simulink model "FM_Bistatic_Radar_Full"  (R2025a)
settings: Solver=VariableStepAuto  StartTime=0.0  StopTime=10.0  RelTol=1e-3
libraries: dspadpt3 x1, commanabbnd3 x1
(part 2 of 3)

== system FM_Bistatic_Radar_Full/Adaptive Filter/Gradiant Adaptive Lattice/50-Stage Lattice Predictor/Stage 41 ==
  note: K Update
  Forward Prediction Error : Inport
  Backward Prediction Error : Inport  Port=2
  K Input : Inport  Port=3
  Delay : Delay  DelayLength=1  InitialCondition=0
  K Update Equation : Subsystem
  Sum : Sum  Inputs=|++
  Sum1 : Sum  Inputs=|++
  Forward Prediction Error Output : Outport
  Backward Prediction Error Output : Outport  Port=2
  K : Outport  Port=3
  wires:
  Sum1/1 -> Backward Prediction Error Output/1
  Delay/1 -> Sum1/2, K Update Equation/2(B I/P)
  Sum/1 -> Forward Prediction Error Output/1
  K Update Equation/2(K) -> K/1, Sum1/1
  K Update Equation/1(*K (K conjugate)) -> Sum/2
  Backward Prediction Error/1 -> Delay/1
  Forward Prediction Error/1 -> Sum/1, K Update Equation/1(F I/P)
  K Input/1 -> K Update Equation/3(K I/P)

== system FM_Bistatic_Radar_Full/Adaptive Filter/Gradiant Adaptive Lattice/50-Stage Lattice Predictor/Stage 42 ==
  note: K Update
  Forward Prediction Error : Inport
  Backward Prediction Error : Inport  Port=2
  K Input : Inport  Port=3
  Delay : Delay  DelayLength=1  InitialCondition=0
  K Update Equation : Subsystem
  Sum : Sum  Inputs=|++
  Sum1 : Sum  Inputs=|++
  Forward Prediction Error Output : Outport
  Backward Prediction Error Output : Outport  Port=2
  K : Outport  Port=3
  wires:
  Sum1/1 -> Backward Prediction Error Output/1
  Delay/1 -> Sum1/2, K Update Equation/2(B I/P)
  Sum/1 -> Forward Prediction Error Output/1
  K Update Equation/2(K) -> K/1, Sum1/1
  K Update Equation/1(*K (K conjugate)) -> Sum/2
  Backward Prediction Error/1 -> Delay/1
  Forward Prediction Error/1 -> Sum/1, K Update Equation/1(F I/P)
  K Input/1 -> K Update Equation/3(K I/P)

== system FM_Bistatic_Radar_Full/Adaptive Filter/Gradiant Adaptive Lattice/50-Stage Lattice Predictor/Stage 43 ==
  note: K Update
  Forward Prediction Error : Inport
  Backward Prediction Error : Inport  Port=2
  K Input : Inport  Port=3
  Delay : Delay  DelayLength=1  InitialCondition=0
  K Update Equation : Subsystem
  Sum : Sum  Inputs=|++
  Sum1 : Sum  Inputs=|++
  Forward Prediction Error Output : Outport
  Backward Prediction Error Output : Outport  Port=2
  K : Outport  Port=3
  wires:
  Sum1/1 -> Backward Prediction Error Output/1
  Delay/1 -> Sum1/2, K Update Equation/2(B I/P)
  Sum/1 -> Forward Prediction Error Output/1
  K Update Equation/2(K) -> K/1, Sum1/1
  K Update Equation/1(*K (K conjugate)) -> Sum/2
  Backward Prediction Error/1 -> Delay/1
  Forward Prediction Error/1 -> Sum/1, K Update Equation/1(F I/P)
  K Input/1 -> K Update Equation/3(K I/P)

== system FM_Bistatic_Radar_Full/Adaptive Filter/Gradiant Adaptive Lattice/50-Stage Lattice Predictor/Stage 44 ==
  note: K Update
  Forward Prediction Error : Inport
  Backward Prediction Error : Inport  Port=2
  K Input : Inport  Port=3
  Delay : Delay  DelayLength=1  InitialCondition=0
  K Update Equation : Subsystem
  Sum : Sum  Inputs=|++
  Sum1 : Sum  Inputs=|++
  Forward Prediction Error Output : Outport
  Backward Prediction Error Output : Outport  Port=2
  K : Outport  Port=3
  wires:
  Sum1/1 -> Backward Prediction Error Output/1
  Delay/1 -> Sum1/2, K Update Equation/2(B I/P)
  Sum/1 -> Forward Prediction Error Output/1
  K Update Equation/2(K) -> K/1, Sum1/1
  K Update Equation/1(*K (K conjugate)) -> Sum/2
  Backward Prediction Error/1 -> Delay/1
  Forward Prediction Error/1 -> Sum/1, K Update Equation/1(F I/P)
  K Input/1 -> K Update Equation/3(K I/P)

== system FM_Bistatic_Radar_Full/Adaptive Filter/Gradiant Adaptive Lattice/50-Stage Lattice Predictor/Stage 45 ==
  note: K Update
  Forward Prediction Error : Inport
  Backward Prediction Error : Inport  Port=2
  K Input : Inport  Port=3
  Delay : Delay  DelayLength=1  InitialCondition=0
  K Update Equation : Subsystem
  Sum : Sum  Inputs=|++
  Sum1 : Sum  Inputs=|++
  Forward Prediction Error Output : Outport
  Backward Prediction Error Output : Outport  Port=2
  K : Outport  Port=3
  wires:
  Sum1/1 -> Backward Prediction Error Output/1
  Delay/1 -> Sum1/2, K Update Equation/2(B I/P)
  Sum/1 -> Forward Prediction Error Output/1
  K Update Equation/2(K) -> K/1, Sum1/1
  K Update Equation/1(*K (K conjugate)) -> Sum/2
  Backward Prediction Error/1 -> Delay/1
  Forward Prediction Error/1 -> Sum/1, K Update Equation/1(F I/P)
  K Input/1 -> K Update Equation/3(K I/P)

== system FM_Bistatic_Radar_Full/Adaptive Filter/Gradiant Adaptive Lattice/50-Stage Lattice Predictor/Stage 46 ==
  note: K Update
  Forward Prediction Error : Inport
  Backward Prediction Error : Inport  Port=2
  K Input : Inport  Port=3
  Delay : Delay  DelayLength=1  InitialCondition=0
  K Update Equation : Subsystem
  Sum : Sum  Inputs=|++
  Sum1 : Sum  Inputs=|++
  Forward Prediction Error Output : Outport
  Backward Prediction Error Output : Outport  Port=2
  K : Outport  Port=3
  wires:
  Sum1/1 -> Backward Prediction Error Output/1
  Delay/1 -> Sum1/2, K Update Equation/2(B I/P)
  Sum/1 -> Forward Prediction Error Output/1
  K Update Equation/2(K) -> K/1, Sum1/1
  K Update Equation/1(*K (K conjugate)) -> Sum/2
  Backward Prediction Error/1 -> Delay/1
  Forward Prediction Error/1 -> Sum/1, K Update Equation/1(F I/P)
  K Input/1 -> K Update Equation/3(K I/P)

== system FM_Bistatic_Radar_Full/Adaptive Filter/Gradiant Adaptive Lattice/50-Stage Lattice Predictor/Stage 47 ==
  note: K Update
  Forward Prediction Error : Inport
  Backward Prediction Error : Inport  Port=2
  K Input : Inport  Port=3
  Delay : Delay  DelayLength=1  InitialCondition=0
  K Update Equation : Subsystem
  Sum : Sum  Inputs=|++
  Sum1 : Sum  Inputs=|++
  Forward Prediction Error Output : Outport
  Backward Prediction Error Output : Outport  Port=2
  K : Outport  Port=3
  wires:
  Sum1/1 -> Backward Prediction Error Output/1
  Delay/1 -> Sum1/2, K Update Equation/2(B I/P)
  Sum/1 -> Forward Prediction Error Output/1
  K Update Equation/2(K) -> K/1, Sum1/1
  K Update Equation/1(*K (K conjugate)) -> Sum/2
  Backward Prediction Error/1 -> Delay/1
  Forward Prediction Error/1 -> Sum/1, K Update Equation/1(F I/P)
  K Input/1 -> K Update Equation/3(K I/P)

== system FM_Bistatic_Radar_Full/Adaptive Filter/Gradiant Adaptive Lattice/50-Stage Lattice Predictor/Stage 48 ==
  note: K Update
  Forward Prediction Error : Inport
  Backward Prediction Error : Inport  Port=2
  K Input : Inport  Port=3
  Delay : Delay  DelayLength=1  InitialCondition=0
  K Update Equation : Subsystem
  Sum : Sum  Inputs=|++
  Sum1 : Sum  Inputs=|++
  Forward Prediction Error Output : Outport
  Backward Prediction Error Output : Outport  Port=2
  K : Outport  Port=3
  wires:
  Sum1/1 -> Backward Prediction Error Output/1
  Delay/1 -> Sum1/2, K Update Equation/2(B I/P)
  Sum/1 -> Forward Prediction Error Output/1
  K Update Equation/2(K) -> K/1, Sum1/1
  K Update Equation/1(*K (K conjugate)) -> Sum/2
  Backward Prediction Error/1 -> Delay/1
  Forward Prediction Error/1 -> Sum/1, K Update Equation/1(F I/P)
  K Input/1 -> K Update Equation/3(K I/P)

== system FM_Bistatic_Radar_Full/Adaptive Filter/Gradiant Adaptive Lattice/50-Stage Lattice Predictor/Stage 49 ==
  note: K Update
  Forward Prediction Error : Inport
  Backward Prediction Error : Inport  Port=2
  K Input : Inport  Port=3
  Delay : Delay  DelayLength=1  InitialCondition=0
  K Update Equation : Subsystem
  Sum : Sum  Inputs=|++
  Sum1 : Sum  Inputs=|++
  Forward Prediction Error Output : Outport
  Backward Prediction Error Output : Outport  Port=2
  K : Outport  Port=3
  wires:
  Sum1/1 -> Backward Prediction Error Output/1
  Delay/1 -> Sum1/2, K Update Equation/2(B I/P)
  Sum/1 -> Forward Prediction Error Output/1
  K Update Equation/2(K) -> K/1, Sum1/1
  K Update Equation/1(*K (K conjugate)) -> Sum/2
  Backward Prediction Error/1 -> Delay/1
  Forward Prediction Error/1 -> Sum/1, K Update Equation/1(F I/P)
  K Input/1 -> K Update Equation/3(K I/P)

== system FM_Bistatic_Radar_Full/Adaptive Filter/Gradiant Adaptive Lattice/50-Stage Lattice Predictor/Stage 5 ==
  note: K Update
  Forward Prediction Error : Inport
  Backward Prediction Error : Inport  Port=2
  K Input : Inport  Port=3
  Delay : Delay  DelayLength=1  InitialCondition=0
  K Update Equation : Subsystem
  Sum : Sum  Inputs=|++
  Sum1 : Sum  Inputs=|++
  Forward Prediction Error Output : Outport
  Backward Prediction Error Output : Outport  Port=2
  K : Outport  Port=3
  wires:
  Sum1/1 -> Backward Prediction Error Output/1
  Delay/1 -> Sum1/2, K Update Equation/2(B I/P)
  Sum/1 -> Forward Prediction Error Output/1
  K Update Equation/2(K) -> K/1, Sum1/1
  K Update Equation/1(*K (K conjugate)) -> Sum/2
  Backward Prediction Error/1 -> Delay/1
  Forward Prediction Error/1 -> Sum/1, K Update Equation/1(F I/P)
  K Input/1 -> K Update Equation/3(K I/P)

== system FM_Bistatic_Radar_Full/Adaptive Filter/Gradiant Adaptive Lattice/50-Stage Lattice Predictor/Stage 50 ==
  note: K Update
  Forward Prediction Error : Inport
  Backward Prediction Error : Inport  Port=2
  K Input : Inport  Port=3
  Delay : Delay  DelayLength=1  InitialCondition=0
  K Update Equation : Subsystem
  Sum : Sum  Inputs=|++
  Sum1 : Sum  Inputs=|++
  Forward Prediction Error Output : Outport
  Backward Prediction Error Output : Outport  Port=2
  K : Outport  Port=3
  wires:
  Sum1/1 -> Backward Prediction Error Output/1
  Delay/1 -> Sum1/2, K Update Equation/2(B I/P)
  Sum/1 -> Forward Prediction Error Output/1
  K Update Equation/2(K) -> K/1, Sum1/1
  K Update Equation/1(*K (K conjugate)) -> Sum/2
  Backward Prediction Error/1 -> Delay/1
  Forward Prediction Error/1 -> Sum/1, K Update Equation/1(F I/P)
  K Input/1 -> K Update Equation/3(K I/P)

== system FM_Bistatic_Radar_Full/Adaptive Filter/Gradiant Adaptive Lattice/50-Stage Lattice Predictor/Stage 51 ==
  note: K Update
  Forward Prediction Error : Inport
  Backward Prediction Error : Inport  Port=2
  K Input : Inport  Port=3
  Delay : Delay  DelayLength=1  InitialCondition=0
  K Update Equation : Subsystem
  Sum : Sum  Inputs=|++
  Sum1 : Sum  Inputs=|++
  Forward Prediction Error Output : Outport
  Backward Prediction Error Output : Outport  Port=2
  K : Outport  Port=3
  wires:
  Sum1/1 -> Backward Prediction Error Output/1
  Delay/1 -> Sum1/2, K Update Equation/2(B I/P)
  Sum/1 -> Forward Prediction Error Output/1
  K Update Equation/2(K) -> K/1, Sum1/1
  K Update Equation/1(*K (K conjugate)) -> Sum/2
  Backward Prediction Error/1 -> Delay/1
  Forward Prediction Error/1 -> Sum/1, K Update Equation/1(F I/P)
  K Input/1 -> K Update Equation/3(K I/P)

== system FM_Bistatic_Radar_Full/Adaptive Filter/Gradiant Adaptive Lattice/50-Stage Lattice Predictor/Stage 6 ==
  note: K Update
  Forward Prediction Error : Inport
  Backward Prediction Error : Inport  Port=2
  K Input : Inport  Port=3
  Delay : Delay  DelayLength=1  InitialCondition=0
  K Update Equation : Subsystem
  Sum : Sum  Inputs=|++
  Sum1 : Sum  Inputs=|++
  Forward Prediction Error Output : Outport
  Backward Prediction Error Output : Outport  Port=2
  K : Outport  Port=3
  wires:
  Sum1/1 -> Backward Prediction Error Output/1
  Delay/1 -> Sum1/2, K Update Equation/2(B I/P)
  Sum/1 -> Forward Prediction Error Output/1
  K Update Equation/2(K) -> K/1, Sum1/1
  K Update Equation/1(*K (K conjugate)) -> Sum/2
  Backward Prediction Error/1 -> Delay/1
  Forward Prediction Error/1 -> Sum/1, K Update Equation/1(F I/P)
  K Input/1 -> K Update Equation/3(K I/P)

== system FM_Bistatic_Radar_Full/Adaptive Filter/Gradiant Adaptive Lattice/50-Stage Lattice Predictor/Stage 7 ==
  note: K Update
  Forward Prediction Error : Inport
  Backward Prediction Error : Inport  Port=2
  K Input : Inport  Port=3
  Delay : Delay  DelayLength=1  InitialCondition=0
  K Update Equation : Subsystem
  Sum : Sum  Inputs=|++
  Sum1 : Sum  Inputs=|++
  Forward Prediction Error Output : Outport
  Backward Prediction Error Output : Outport  Port=2
  K : Outport  Port=3
  wires:
  Sum1/1 -> Backward Prediction Error Output/1
  Delay/1 -> Sum1/2, K Update Equation/2(B I/P)
  Sum/1 -> Forward Prediction Error Output/1
  K Update Equation/2(K) -> K/1, Sum1/1
  K Update Equation/1(*K (K conjugate)) -> Sum/2
  Backward Prediction Error/1 -> Delay/1
  Forward Prediction Error/1 -> Sum/1, K Update Equation/1(F I/P)
  K Input/1 -> K Update Equation/3(K I/P)

== system FM_Bistatic_Radar_Full/Adaptive Filter/Gradiant Adaptive Lattice/50-Stage Lattice Predictor/Stage 8 ==
  note: K Update
  Forward Prediction Error : Inport
  Backward Prediction Error : Inport  Port=2
  K Input : Inport  Port=3
  Delay : Delay  DelayLength=1  InitialCondition=0
  K Update Equation : Subsystem
  Sum : Sum  Inputs=|++
  Sum1 : Sum  Inputs=|++
  Forward Prediction Error Output : Outport
  Backward Prediction Error Output : Outport  Port=2
  K : Outport  Port=3
  wires:
  Sum1/1 -> Backward Prediction Error Output/1
  Delay/1 -> Sum1/2, K Update Equation/2(B I/P)
  Sum/1 -> Forward Prediction Error Output/1
  K Update Equation/2(K) -> K/1, Sum1/1
  K Update Equation/1(*K (K conjugate)) -> Sum/2
  Backward Prediction Error/1 -> Delay/1
  Forward Prediction Error/1 -> Sum/1, K Update Equation/1(F I/P)
  K Input/1 -> K Update Equation/3(K I/P)

== system FM_Bistatic_Radar_Full/Adaptive Filter/Gradiant Adaptive Lattice/50-Stage Lattice Predictor/Stage 9 ==
  note: K Update
  Forward Prediction Error : Inport
  Backward Prediction Error : Inport  Port=2
  K Input : Inport  Port=3
  Delay : Delay  DelayLength=1  InitialCondition=0
  K Update Equation : Subsystem
  Sum : Sum  Inputs=|++
  Sum1 : Sum  Inputs=|++
  Forward Prediction Error Output : Outport
  Backward Prediction Error Output : Outport  Port=2
  K : Outport  Port=3
  wires:
  Sum1/1 -> Backward Prediction Error Output/1
  Delay/1 -> Sum1/2, K Update Equation/2(B I/P)
  Sum/1 -> Forward Prediction Error Output/1
  K Update Equation/2(K) -> K/1, Sum1/1
  K Update Equation/1(*K (K conjugate)) -> Sum/2
  Backward Prediction Error/1 -> Delay/1
  Forward Prediction Error/1 -> Sum/1, K Update Equation/1(F I/P)
  K Input/1 -> K Update Equation/3(K I/P)

== system FM_Bistatic_Radar_Full/Adaptive Filter/Gradiant Adaptive Lattice/50-Stage Lattice Predictor/Stage 1/K Update Equation ==
  F I/P : Inport
  B I/P : Inport  Port=2
  Conjugate : Math  Operator=conj  SignedPower=on  RndMeth=Zero
  Conjugate1 : Math  Operator=conj  SignedPower=on  RndMeth=Zero
  Constant : Constant  Value=0.01
  Dot Product : DotProduct  OutDataTypeStr=Inherit: Inherit via internal rule
  Dot Product1 : DotProduct  OutDataTypeStr=Inherit: Inherit via internal rule
  Subtract : Sum  Inputs=+-
  *K (K conjugate) : Outport
  K : Outport  Port=2
  wires:
  F I/P/1 -> Subtract/1, Dot Product/1
  B I/P/1 -> Conjugate/1
  Conjugate/1 -> Dot Product/2
  Constant/1 -> Dot Product1/2
  Dot Product/1 -> Dot Product1/1
  Conjugate1/1 -> *K (K conjugate)/1
  Dot Product1/1 -> Subtract/2
  Subtract/1 -> K/1, Conjugate1/1

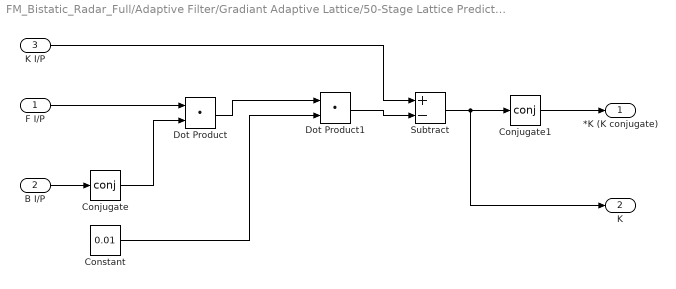
== system FM_Bistatic_Radar_Full/Adaptive Filter/Gradiant Adaptive Lattice/50-Stage Lattice Predictor/Stage 10/K Update Equation ==
  F I/P : Inport
  B I/P : Inport  Port=2
  K I/P : Inport  Port=3
  Conjugate : Math  Operator=conj  SignedPower=on  RndMeth=Zero
  Conjugate1 : Math  Operator=conj  SignedPower=on  RndMeth=Zero
  Constant : Constant  Value=0.01
  Dot Product : DotProduct  OutDataTypeStr=Inherit: Inherit via internal rule
  Dot Product1 : DotProduct  OutDataTypeStr=Inherit: Inherit via internal rule
  Subtract : Sum  Inputs=+-
  *K (K conjugate) : Outport
  K : Outport  Port=2
  wires:
  F I/P/1 -> Dot Product/1
  B I/P/1 -> Conjugate/1
  Conjugate/1 -> Dot Product/2
  Constant/1 -> Dot Product1/2
  Dot Product/1 -> Dot Product1/1
  Conjugate1/1 -> *K (K conjugate)/1
  Dot Product1/1 -> Subtract/2
  Subtract/1 -> K/1, Conjugate1/1
  K I/P/1 -> Subtract/1

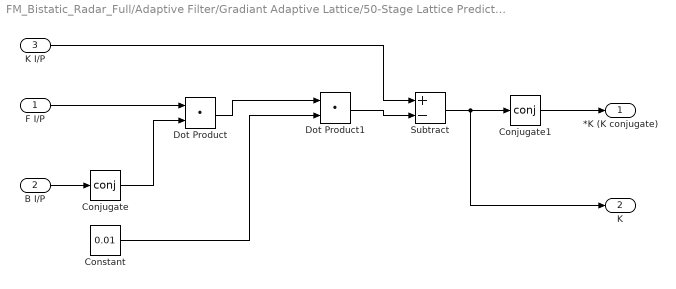
== system FM_Bistatic_Radar_Full/Adaptive Filter/Gradiant Adaptive Lattice/50-Stage Lattice Predictor/Stage 11/K Update Equation ==
  F I/P : Inport
  B I/P : Inport  Port=2
  K I/P : Inport  Port=3
  Conjugate : Math  Operator=conj  SignedPower=on  RndMeth=Zero
  Conjugate1 : Math  Operator=conj  SignedPower=on  RndMeth=Zero
  Constant : Constant  Value=0.01
  Dot Product : DotProduct  OutDataTypeStr=Inherit: Inherit via internal rule
  Dot Product1 : DotProduct  OutDataTypeStr=Inherit: Inherit via internal rule
  Subtract : Sum  Inputs=+-
  *K (K conjugate) : Outport
  K : Outport  Port=2
  wires:
  F I/P/1 -> Dot Product/1
  B I/P/1 -> Conjugate/1
  Conjugate/1 -> Dot Product/2
  Constant/1 -> Dot Product1/2
  Dot Product/1 -> Dot Product1/1
  Conjugate1/1 -> *K (K conjugate)/1
  Dot Product1/1 -> Subtract/2
  Subtract/1 -> K/1, Conjugate1/1
  K I/P/1 -> Subtract/1

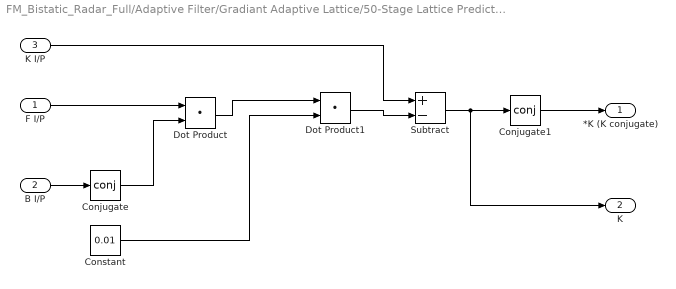
== system FM_Bistatic_Radar_Full/Adaptive Filter/Gradiant Adaptive Lattice/50-Stage Lattice Predictor/Stage 12/K Update Equation ==
  F I/P : Inport
  B I/P : Inport  Port=2
  K I/P : Inport  Port=3
  Conjugate : Math  Operator=conj  SignedPower=on  RndMeth=Zero
  Conjugate1 : Math  Operator=conj  SignedPower=on  RndMeth=Zero
  Constant : Constant  Value=0.01
  Dot Product : DotProduct  OutDataTypeStr=Inherit: Inherit via internal rule
  Dot Product1 : DotProduct  OutDataTypeStr=Inherit: Inherit via internal rule
  Subtract : Sum  Inputs=+-
  *K (K conjugate) : Outport
  K : Outport  Port=2
  wires:
  F I/P/1 -> Dot Product/1
  B I/P/1 -> Conjugate/1
  Conjugate/1 -> Dot Product/2
  Constant/1 -> Dot Product1/2
  Dot Product/1 -> Dot Product1/1
  Conjugate1/1 -> *K (K conjugate)/1
  Dot Product1/1 -> Subtract/2
  Subtract/1 -> K/1, Conjugate1/1
  K I/P/1 -> Subtract/1

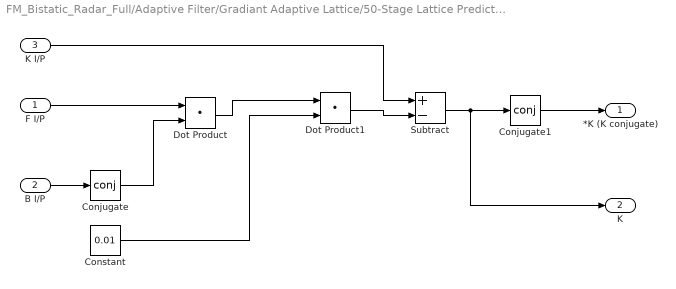
== system FM_Bistatic_Radar_Full/Adaptive Filter/Gradiant Adaptive Lattice/50-Stage Lattice Predictor/Stage 13/K Update Equation ==
  F I/P : Inport
  B I/P : Inport  Port=2
  K I/P : Inport  Port=3
  Conjugate : Math  Operator=conj  SignedPower=on  RndMeth=Zero
  Conjugate1 : Math  Operator=conj  SignedPower=on  RndMeth=Zero
  Constant : Constant  Value=0.01
  Dot Product : DotProduct  OutDataTypeStr=Inherit: Inherit via internal rule
  Dot Product1 : DotProduct  OutDataTypeStr=Inherit: Inherit via internal rule
  Subtract : Sum  Inputs=+-
  *K (K conjugate) : Outport
  K : Outport  Port=2
  wires:
  F I/P/1 -> Dot Product/1
  B I/P/1 -> Conjugate/1
  Conjugate/1 -> Dot Product/2
  Constant/1 -> Dot Product1/2
  Dot Product/1 -> Dot Product1/1
  Conjugate1/1 -> *K (K conjugate)/1
  Dot Product1/1 -> Subtract/2
  Subtract/1 -> K/1, Conjugate1/1
  K I/P/1 -> Subtract/1

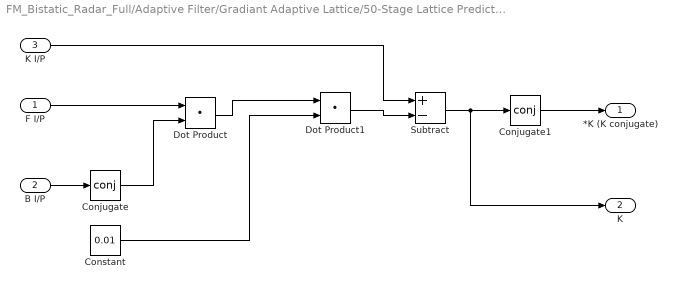
== system FM_Bistatic_Radar_Full/Adaptive Filter/Gradiant Adaptive Lattice/50-Stage Lattice Predictor/Stage 14/K Update Equation ==
  F I/P : Inport
  B I/P : Inport  Port=2
  K I/P : Inport  Port=3
  Conjugate : Math  Operator=conj  SignedPower=on  RndMeth=Zero
  Conjugate1 : Math  Operator=conj  SignedPower=on  RndMeth=Zero
  Constant : Constant  Value=0.01
  Dot Product : DotProduct  OutDataTypeStr=Inherit: Inherit via internal rule
  Dot Product1 : DotProduct  OutDataTypeStr=Inherit: Inherit via internal rule
  Subtract : Sum  Inputs=+-
  *K (K conjugate) : Outport
  K : Outport  Port=2
  wires:
  F I/P/1 -> Dot Product/1
  B I/P/1 -> Conjugate/1
  Conjugate/1 -> Dot Product/2
  Constant/1 -> Dot Product1/2
  Dot Product/1 -> Dot Product1/1
  Conjugate1/1 -> *K (K conjugate)/1
  Dot Product1/1 -> Subtract/2
  Subtract/1 -> K/1, Conjugate1/1
  K I/P/1 -> Subtract/1

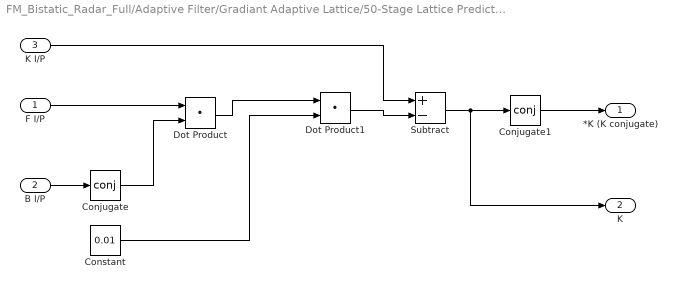
== system FM_Bistatic_Radar_Full/Adaptive Filter/Gradiant Adaptive Lattice/50-Stage Lattice Predictor/Stage 15/K Update Equation ==
  F I/P : Inport
  B I/P : Inport  Port=2
  K I/P : Inport  Port=3
  Conjugate : Math  Operator=conj  SignedPower=on  RndMeth=Zero
  Conjugate1 : Math  Operator=conj  SignedPower=on  RndMeth=Zero
  Constant : Constant  Value=0.01
  Dot Product : DotProduct  OutDataTypeStr=Inherit: Inherit via internal rule
  Dot Product1 : DotProduct  OutDataTypeStr=Inherit: Inherit via internal rule
  Subtract : Sum  Inputs=+-
  *K (K conjugate) : Outport
  K : Outport  Port=2
  wires:
  F I/P/1 -> Dot Product/1
  B I/P/1 -> Conjugate/1
  Conjugate/1 -> Dot Product/2
  Constant/1 -> Dot Product1/2
  Dot Product/1 -> Dot Product1/1
  Conjugate1/1 -> *K (K conjugate)/1
  Dot Product1/1 -> Subtract/2
  Subtract/1 -> K/1, Conjugate1/1
  K I/P/1 -> Subtract/1

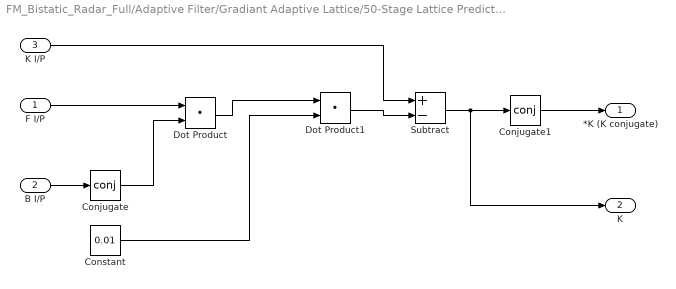
== system FM_Bistatic_Radar_Full/Adaptive Filter/Gradiant Adaptive Lattice/50-Stage Lattice Predictor/Stage 16/K Update Equation ==
  F I/P : Inport
  B I/P : Inport  Port=2
  K I/P : Inport  Port=3
  Conjugate : Math  Operator=conj  SignedPower=on  RndMeth=Zero
  Conjugate1 : Math  Operator=conj  SignedPower=on  RndMeth=Zero
  Constant : Constant  Value=0.01
  Dot Product : DotProduct  OutDataTypeStr=Inherit: Inherit via internal rule
  Dot Product1 : DotProduct  OutDataTypeStr=Inherit: Inherit via internal rule
  Subtract : Sum  Inputs=+-
  *K (K conjugate) : Outport
  K : Outport  Port=2
  wires:
  F I/P/1 -> Dot Product/1
  B I/P/1 -> Conjugate/1
  Conjugate/1 -> Dot Product/2
  Constant/1 -> Dot Product1/2
  Dot Product/1 -> Dot Product1/1
  Conjugate1/1 -> *K (K conjugate)/1
  Dot Product1/1 -> Subtract/2
  Subtract/1 -> K/1, Conjugate1/1
  K I/P/1 -> Subtract/1

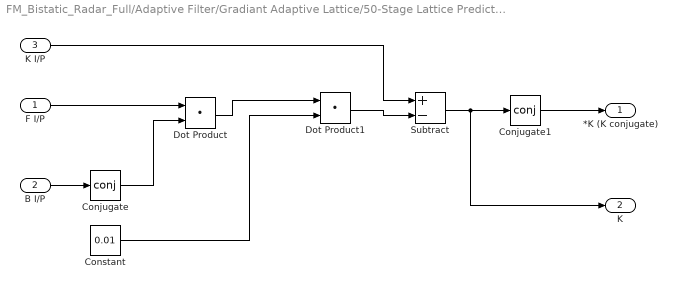
== system FM_Bistatic_Radar_Full/Adaptive Filter/Gradiant Adaptive Lattice/50-Stage Lattice Predictor/Stage 17/K Update Equation ==
  F I/P : Inport
  B I/P : Inport  Port=2
  K I/P : Inport  Port=3
  Conjugate : Math  Operator=conj  SignedPower=on  RndMeth=Zero
  Conjugate1 : Math  Operator=conj  SignedPower=on  RndMeth=Zero
  Constant : Constant  Value=0.01
  Dot Product : DotProduct  OutDataTypeStr=Inherit: Inherit via internal rule
  Dot Product1 : DotProduct  OutDataTypeStr=Inherit: Inherit via internal rule
  Subtract : Sum  Inputs=+-
  *K (K conjugate) : Outport
  K : Outport  Port=2
  wires:
  F I/P/1 -> Dot Product/1
  B I/P/1 -> Conjugate/1
  Conjugate/1 -> Dot Product/2
  Constant/1 -> Dot Product1/2
  Dot Product/1 -> Dot Product1/1
  Conjugate1/1 -> *K (K conjugate)/1
  Dot Product1/1 -> Subtract/2
  Subtract/1 -> K/1, Conjugate1/1
  K I/P/1 -> Subtract/1

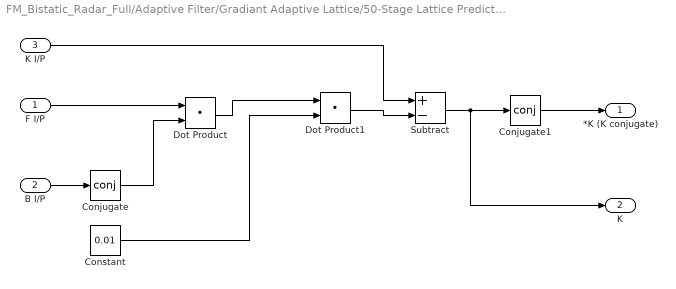
== system FM_Bistatic_Radar_Full/Adaptive Filter/Gradiant Adaptive Lattice/50-Stage Lattice Predictor/Stage 18/K Update Equation ==
  F I/P : Inport
  B I/P : Inport  Port=2
  K I/P : Inport  Port=3
  Conjugate : Math  Operator=conj  SignedPower=on  RndMeth=Zero
  Conjugate1 : Math  Operator=conj  SignedPower=on  RndMeth=Zero
  Constant : Constant  Value=0.01
  Dot Product : DotProduct  OutDataTypeStr=Inherit: Inherit via internal rule
  Dot Product1 : DotProduct  OutDataTypeStr=Inherit: Inherit via internal rule
  Subtract : Sum  Inputs=+-
  *K (K conjugate) : Outport
  K : Outport  Port=2
  wires:
  F I/P/1 -> Dot Product/1
  B I/P/1 -> Conjugate/1
  Conjugate/1 -> Dot Product/2
  Constant/1 -> Dot Product1/2
  Dot Product/1 -> Dot Product1/1
  Conjugate1/1 -> *K (K conjugate)/1
  Dot Product1/1 -> Subtract/2
  Subtract/1 -> K/1, Conjugate1/1
  K I/P/1 -> Subtract/1

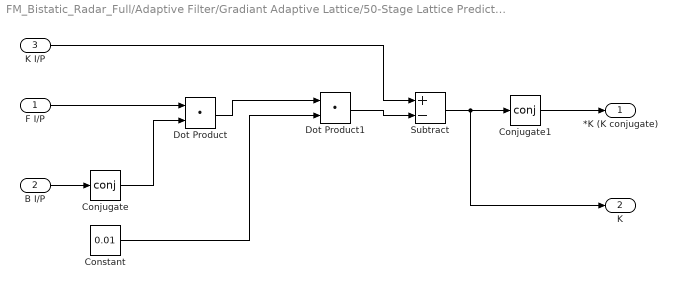
== system FM_Bistatic_Radar_Full/Adaptive Filter/Gradiant Adaptive Lattice/50-Stage Lattice Predictor/Stage 19/K Update Equation ==
  F I/P : Inport
  B I/P : Inport  Port=2
  K I/P : Inport  Port=3
  Conjugate : Math  Operator=conj  SignedPower=on  RndMeth=Zero
  Conjugate1 : Math  Operator=conj  SignedPower=on  RndMeth=Zero
  Constant : Constant  Value=0.01
  Dot Product : DotProduct  OutDataTypeStr=Inherit: Inherit via internal rule
  Dot Product1 : DotProduct  OutDataTypeStr=Inherit: Inherit via internal rule
  Subtract : Sum  Inputs=+-
  *K (K conjugate) : Outport
  K : Outport  Port=2
  wires:
  F I/P/1 -> Dot Product/1
  B I/P/1 -> Conjugate/1
  Conjugate/1 -> Dot Product/2
  Constant/1 -> Dot Product1/2
  Dot Product/1 -> Dot Product1/1
  Conjugate1/1 -> *K (K conjugate)/1
  Dot Product1/1 -> Subtract/2
  Subtract/1 -> K/1, Conjugate1/1
  K I/P/1 -> Subtract/1

== system FM_Bistatic_Radar_Full/Adaptive Filter/Gradiant Adaptive Lattice/50-Stage Lattice Predictor/Stage 2/K Update Equation ==
  F I/P : Inport
  B I/P : Inport  Port=2
  K I/P : Inport  Port=3
  Conjugate : Math  Operator=conj  SignedPower=on  RndMeth=Zero
  Conjugate1 : Math  Operator=conj  SignedPower=on  RndMeth=Zero
  Constant : Constant  Value=0.01
  Dot Product : DotProduct  OutDataTypeStr=Inherit: Inherit via internal rule
  Dot Product1 : DotProduct  OutDataTypeStr=Inherit: Inherit via internal rule
  Subtract : Sum  Inputs=+-
  *K (K conjugate) : Outport
  K : Outport  Port=2
  wires:
  F I/P/1 -> Dot Product/1
  B I/P/1 -> Conjugate/1
  Conjugate/1 -> Dot Product/2
  Constant/1 -> Dot Product1/2
  Dot Product/1 -> Dot Product1/1
  Conjugate1/1 -> *K (K conjugate)/1
  Dot Product1/1 -> Subtract/2
  Subtract/1 -> K/1, Conjugate1/1
  K I/P/1 -> Subtract/1

== system FM_Bistatic_Radar_Full/Adaptive Filter/Gradiant Adaptive Lattice/50-Stage Lattice Predictor/Stage 20/K Update Equation ==
  F I/P : Inport
  B I/P : Inport  Port=2
  K I/P : Inport  Port=3
  Conjugate : Math  Operator=conj  SignedPower=on  RndMeth=Zero
  Conjugate1 : Math  Operator=conj  SignedPower=on  RndMeth=Zero
  Constant : Constant  Value=0.01
  Dot Product : DotProduct  OutDataTypeStr=Inherit: Inherit via internal rule
  Dot Product1 : DotProduct  OutDataTypeStr=Inherit: Inherit via internal rule
  Subtract : Sum  Inputs=+-
  *K (K conjugate) : Outport
  K : Outport  Port=2
  wires:
  F I/P/1 -> Dot Product/1
  B I/P/1 -> Conjugate/1
  Conjugate/1 -> Dot Product/2
  Constant/1 -> Dot Product1/2
  Dot Product/1 -> Dot Product1/1
  Conjugate1/1 -> *K (K conjugate)/1
  Dot Product1/1 -> Subtract/2
  Subtract/1 -> K/1, Conjugate1/1
  K I/P/1 -> Subtract/1

== system FM_Bistatic_Radar_Full/Adaptive Filter/Gradiant Adaptive Lattice/50-Stage Lattice Predictor/Stage 21/K Update Equation ==
  F I/P : Inport
  B I/P : Inport  Port=2
  K I/P : Inport  Port=3
  Conjugate : Math  Operator=conj  SignedPower=on  RndMeth=Zero
  Conjugate1 : Math  Operator=conj  SignedPower=on  RndMeth=Zero
  Constant : Constant  Value=0.01
  Dot Product : DotProduct  OutDataTypeStr=Inherit: Inherit via internal rule
  Dot Product1 : DotProduct  OutDataTypeStr=Inherit: Inherit via internal rule
  Subtract : Sum  Inputs=+-
  *K (K conjugate) : Outport
  K : Outport  Port=2
  wires:
  F I/P/1 -> Dot Product/1
  B I/P/1 -> Conjugate/1
  Conjugate/1 -> Dot Product/2
  Constant/1 -> Dot Product1/2
  Dot Product/1 -> Dot Product1/1
  Conjugate1/1 -> *K (K conjugate)/1
  Dot Product1/1 -> Subtract/2
  Subtract/1 -> K/1, Conjugate1/1
  K I/P/1 -> Subtract/1

== system FM_Bistatic_Radar_Full/Adaptive Filter/Gradiant Adaptive Lattice/50-Stage Lattice Predictor/Stage 22/K Update Equation ==
  F I/P : Inport
  B I/P : Inport  Port=2
  K I/P : Inport  Port=3
  Conjugate : Math  Operator=conj  SignedPower=on  RndMeth=Zero
  Conjugate1 : Math  Operator=conj  SignedPower=on  RndMeth=Zero
  Constant : Constant  Value=0.01
  Dot Product : DotProduct  OutDataTypeStr=Inherit: Inherit via internal rule
  Dot Product1 : DotProduct  OutDataTypeStr=Inherit: Inherit via internal rule
  Subtract : Sum  Inputs=+-
  *K (K conjugate) : Outport
  K : Outport  Port=2
  wires:
  F I/P/1 -> Dot Product/1
  B I/P/1 -> Conjugate/1
  Conjugate/1 -> Dot Product/2
  Constant/1 -> Dot Product1/2
  Dot Product/1 -> Dot Product1/1
  Conjugate1/1 -> *K (K conjugate)/1
  Dot Product1/1 -> Subtract/2
  Subtract/1 -> K/1, Conjugate1/1
  K I/P/1 -> Subtract/1

== system FM_Bistatic_Radar_Full/Adaptive Filter/Gradiant Adaptive Lattice/50-Stage Lattice Predictor/Stage 23/K Update Equation ==
  F I/P : Inport
  B I/P : Inport  Port=2
  K I/P : Inport  Port=3
  Conjugate : Math  Operator=conj  SignedPower=on  RndMeth=Zero
  Conjugate1 : Math  Operator=conj  SignedPower=on  RndMeth=Zero
  Constant : Constant  Value=0.01
  Dot Product : DotProduct  OutDataTypeStr=Inherit: Inherit via internal rule
  Dot Product1 : DotProduct  OutDataTypeStr=Inherit: Inherit via internal rule
  Subtract : Sum  Inputs=+-
  *K (K conjugate) : Outport
  K : Outport  Port=2
  wires:
  F I/P/1 -> Dot Product/1
  B I/P/1 -> Conjugate/1
  Conjugate/1 -> Dot Product/2
  Constant/1 -> Dot Product1/2
  Dot Product/1 -> Dot Product1/1
  Conjugate1/1 -> *K (K conjugate)/1
  Dot Product1/1 -> Subtract/2
  Subtract/1 -> K/1, Conjugate1/1
  K I/P/1 -> Subtract/1

== system FM_Bistatic_Radar_Full/Adaptive Filter/Gradiant Adaptive Lattice/50-Stage Lattice Predictor/Stage 24/K Update Equation ==
  F I/P : Inport
  B I/P : Inport  Port=2
  K I/P : Inport  Port=3
  Conjugate : Math  Operator=conj  SignedPower=on  RndMeth=Zero
  Conjugate1 : Math  Operator=conj  SignedPower=on  RndMeth=Zero
  Constant : Constant  Value=0.01
  Dot Product : DotProduct  OutDataTypeStr=Inherit: Inherit via internal rule
  Dot Product1 : DotProduct  OutDataTypeStr=Inherit: Inherit via internal rule
  Subtract : Sum  Inputs=+-
  *K (K conjugate) : Outport
  K : Outport  Port=2
  wires:
  F I/P/1 -> Dot Product/1
  B I/P/1 -> Conjugate/1
  Conjugate/1 -> Dot Product/2
  Constant/1 -> Dot Product1/2
  Dot Product/1 -> Dot Product1/1
  Conjugate1/1 -> *K (K conjugate)/1
  Dot Product1/1 -> Subtract/2
  Subtract/1 -> K/1, Conjugate1/1
  K I/P/1 -> Subtract/1

== system FM_Bistatic_Radar_Full/Adaptive Filter/Gradiant Adaptive Lattice/50-Stage Lattice Predictor/Stage 25/K Update Equation ==
  F I/P : Inport
  B I/P : Inport  Port=2
  K I/P : Inport  Port=3
  Conjugate : Math  Operator=conj  SignedPower=on  RndMeth=Zero
  Conjugate1 : Math  Operator=conj  SignedPower=on  RndMeth=Zero
  Constant : Constant  Value=0.01
  Dot Product : DotProduct  OutDataTypeStr=Inherit: Inherit via internal rule
  Dot Product1 : DotProduct  OutDataTypeStr=Inherit: Inherit via internal rule
  Subtract : Sum  Inputs=+-
  *K (K conjugate) : Outport
  K : Outport  Port=2
  wires:
  F I/P/1 -> Dot Product/1
  B I/P/1 -> Conjugate/1
  Conjugate/1 -> Dot Product/2
  Constant/1 -> Dot Product1/2
  Dot Product/1 -> Dot Product1/1
  Conjugate1/1 -> *K (K conjugate)/1
  Dot Product1/1 -> Subtract/2
  Subtract/1 -> K/1, Conjugate1/1
  K I/P/1 -> Subtract/1

== system FM_Bistatic_Radar_Full/Adaptive Filter/Gradiant Adaptive Lattice/50-Stage Lattice Predictor/Stage 26/K Update Equation ==
  F I/P : Inport
  B I/P : Inport  Port=2
  K I/P : Inport  Port=3
  Conjugate : Math  Operator=conj  SignedPower=on  RndMeth=Zero
  Conjugate1 : Math  Operator=conj  SignedPower=on  RndMeth=Zero
  Constant : Constant  Value=0.01
  Dot Product : DotProduct  OutDataTypeStr=Inherit: Inherit via internal rule
  Dot Product1 : DotProduct  OutDataTypeStr=Inherit: Inherit via internal rule
  Subtract : Sum  Inputs=+-
  *K (K conjugate) : Outport
  K : Outport  Port=2
  wires:
  F I/P/1 -> Dot Product/1
  B I/P/1 -> Conjugate/1
  Conjugate/1 -> Dot Product/2
  Constant/1 -> Dot Product1/2
  Dot Product/1 -> Dot Product1/1
  Conjugate1/1 -> *K (K conjugate)/1
  Dot Product1/1 -> Subtract/2
  Subtract/1 -> K/1, Conjugate1/1
  K I/P/1 -> Subtract/1

== system FM_Bistatic_Radar_Full/Adaptive Filter/Gradiant Adaptive Lattice/50-Stage Lattice Predictor/Stage 27/K Update Equation ==
  F I/P : Inport
  B I/P : Inport  Port=2
  K I/P : Inport  Port=3
  Conjugate : Math  Operator=conj  SignedPower=on  RndMeth=Zero
  Conjugate1 : Math  Operator=conj  SignedPower=on  RndMeth=Zero
  Constant : Constant  Value=0.01
  Dot Product : DotProduct  OutDataTypeStr=Inherit: Inherit via internal rule
  Dot Product1 : DotProduct  OutDataTypeStr=Inherit: Inherit via internal rule
  Subtract : Sum  Inputs=+-
  *K (K conjugate) : Outport
  K : Outport  Port=2
  wires:
  F I/P/1 -> Dot Product/1
  B I/P/1 -> Conjugate/1
  Conjugate/1 -> Dot Product/2
  Constant/1 -> Dot Product1/2
  Dot Product/1 -> Dot Product1/1
  Conjugate1/1 -> *K (K conjugate)/1
  Dot Product1/1 -> Subtract/2
  Subtract/1 -> K/1, Conjugate1/1
  K I/P/1 -> Subtract/1

== system FM_Bistatic_Radar_Full/Adaptive Filter/Gradiant Adaptive Lattice/50-Stage Lattice Predictor/Stage 28/K Update Equation ==
  F I/P : Inport
  B I/P : Inport  Port=2
  K I/P : Inport  Port=3
  Conjugate : Math  Operator=conj  SignedPower=on  RndMeth=Zero
  Conjugate1 : Math  Operator=conj  SignedPower=on  RndMeth=Zero
  Constant : Constant  Value=0.01
  Dot Product : DotProduct  OutDataTypeStr=Inherit: Inherit via internal rule
  Dot Product1 : DotProduct  OutDataTypeStr=Inherit: Inherit via internal rule
  Subtract : Sum  Inputs=+-
  *K (K conjugate) : Outport
  K : Outport  Port=2
  wires:
  F I/P/1 -> Dot Product/1
  B I/P/1 -> Conjugate/1
  Conjugate/1 -> Dot Product/2
  Constant/1 -> Dot Product1/2
  Dot Product/1 -> Dot Product1/1
  Conjugate1/1 -> *K (K conjugate)/1
  Dot Product1/1 -> Subtract/2
  Subtract/1 -> K/1, Conjugate1/1
  K I/P/1 -> Subtract/1

== system FM_Bistatic_Radar_Full/Adaptive Filter/Gradiant Adaptive Lattice/50-Stage Lattice Predictor/Stage 29/K Update Equation ==
  F I/P : Inport
  B I/P : Inport  Port=2
  K I/P : Inport  Port=3
  Conjugate : Math  Operator=conj  SignedPower=on  RndMeth=Zero
  Conjugate1 : Math  Operator=conj  SignedPower=on  RndMeth=Zero
  Constant : Constant  Value=0.01
  Dot Product : DotProduct  OutDataTypeStr=Inherit: Inherit via internal rule
  Dot Product1 : DotProduct  OutDataTypeStr=Inherit: Inherit via internal rule
  Subtract : Sum  Inputs=+-
  *K (K conjugate) : Outport
  K : Outport  Port=2
  wires:
  F I/P/1 -> Dot Product/1
  B I/P/1 -> Conjugate/1
  Conjugate/1 -> Dot Product/2
  Constant/1 -> Dot Product1/2
  Dot Product/1 -> Dot Product1/1
  Conjugate1/1 -> *K (K conjugate)/1
  Dot Product1/1 -> Subtract/2
  Subtract/1 -> K/1, Conjugate1/1
  K I/P/1 -> Subtract/1

== system FM_Bistatic_Radar_Full/Adaptive Filter/Gradiant Adaptive Lattice/50-Stage Lattice Predictor/Stage 3/K Update Equation ==
  F I/P : Inport
  B I/P : Inport  Port=2
  K I/P : Inport  Port=3
  Conjugate : Math  Operator=conj  SignedPower=on  RndMeth=Zero
  Conjugate1 : Math  Operator=conj  SignedPower=on  RndMeth=Zero
  Constant : Constant  Value=0.01
  Dot Product : DotProduct  OutDataTypeStr=Inherit: Inherit via internal rule
  Dot Product1 : DotProduct  OutDataTypeStr=Inherit: Inherit via internal rule
  Subtract : Sum  Inputs=+-
  *K (K conjugate) : Outport
  K : Outport  Port=2
  wires:
  F I/P/1 -> Dot Product/1
  B I/P/1 -> Conjugate/1
  Conjugate/1 -> Dot Product/2
  Constant/1 -> Dot Product1/2
  Dot Product/1 -> Dot Product1/1
  Conjugate1/1 -> *K (K conjugate)/1
  Dot Product1/1 -> Subtract/2
  Subtract/1 -> K/1, Conjugate1/1
  K I/P/1 -> Subtract/1

== system FM_Bistatic_Radar_Full/Adaptive Filter/Gradiant Adaptive Lattice/50-Stage Lattice Predictor/Stage 30/K Update Equation ==
  F I/P : Inport
  B I/P : Inport  Port=2
  K I/P : Inport  Port=3
  Conjugate : Math  Operator=conj  SignedPower=on  RndMeth=Zero
  Conjugate1 : Math  Operator=conj  SignedPower=on  RndMeth=Zero
  Constant : Constant  Value=0.01
  Dot Product : DotProduct  OutDataTypeStr=Inherit: Inherit via internal rule
  Dot Product1 : DotProduct  OutDataTypeStr=Inherit: Inherit via internal rule
  Subtract : Sum  Inputs=+-
  *K (K conjugate) : Outport
  K : Outport  Port=2
  wires:
  F I/P/1 -> Dot Product/1
  B I/P/1 -> Conjugate/1
  Conjugate/1 -> Dot Product/2
  Constant/1 -> Dot Product1/2
  Dot Product/1 -> Dot Product1/1
  Conjugate1/1 -> *K (K conjugate)/1
  Dot Product1/1 -> Subtract/2
  Subtract/1 -> K/1, Conjugate1/1
  K I/P/1 -> Subtract/1

== system FM_Bistatic_Radar_Full/Adaptive Filter/Gradiant Adaptive Lattice/50-Stage Lattice Predictor/Stage 31/K Update Equation ==
  F I/P : Inport
  B I/P : Inport  Port=2
  K I/P : Inport  Port=3
  Conjugate : Math  Operator=conj  SignedPower=on  RndMeth=Zero
  Conjugate1 : Math  Operator=conj  SignedPower=on  RndMeth=Zero
  Constant : Constant  Value=0.01
  Dot Product : DotProduct  OutDataTypeStr=Inherit: Inherit via internal rule
  Dot Product1 : DotProduct  OutDataTypeStr=Inherit: Inherit via internal rule
  Subtract : Sum  Inputs=+-
  *K (K conjugate) : Outport
  K : Outport  Port=2
  wires:
  F I/P/1 -> Dot Product/1
  B I/P/1 -> Conjugate/1
  Conjugate/1 -> Dot Product/2
  Constant/1 -> Dot Product1/2
  Dot Product/1 -> Dot Product1/1
  Conjugate1/1 -> *K (K conjugate)/1
  Dot Product1/1 -> Subtract/2
  Subtract/1 -> K/1, Conjugate1/1
  K I/P/1 -> Subtract/1

== system FM_Bistatic_Radar_Full/Adaptive Filter/Gradiant Adaptive Lattice/50-Stage Lattice Predictor/Stage 32/K Update Equation ==
  F I/P : Inport
  B I/P : Inport  Port=2
  K I/P : Inport  Port=3
  Conjugate : Math  Operator=conj  SignedPower=on  RndMeth=Zero
  Conjugate1 : Math  Operator=conj  SignedPower=on  RndMeth=Zero
  Constant : Constant  Value=0.01
  Dot Product : DotProduct  OutDataTypeStr=Inherit: Inherit via internal rule
  Dot Product1 : DotProduct  OutDataTypeStr=Inherit: Inherit via internal rule
  Subtract : Sum  Inputs=+-
  *K (K conjugate) : Outport
  K : Outport  Port=2
  wires:
  F I/P/1 -> Dot Product/1
  B I/P/1 -> Conjugate/1
  Conjugate/1 -> Dot Product/2
  Constant/1 -> Dot Product1/2
  Dot Product/1 -> Dot Product1/1
  Conjugate1/1 -> *K (K conjugate)/1
  Dot Product1/1 -> Subtract/2
  Subtract/1 -> K/1, Conjugate1/1
  K I/P/1 -> Subtract/1

== system FM_Bistatic_Radar_Full/Adaptive Filter/Gradiant Adaptive Lattice/50-Stage Lattice Predictor/Stage 33/K Update Equation ==
  F I/P : Inport
  B I/P : Inport  Port=2
  K I/P : Inport  Port=3
  Conjugate : Math  Operator=conj  SignedPower=on  RndMeth=Zero
  Conjugate1 : Math  Operator=conj  SignedPower=on  RndMeth=Zero
  Constant : Constant  Value=0.01
  Dot Product : DotProduct  OutDataTypeStr=Inherit: Inherit via internal rule
  Dot Product1 : DotProduct  OutDataTypeStr=Inherit: Inherit via internal rule
  Subtract : Sum  Inputs=+-
  *K (K conjugate) : Outport
  K : Outport  Port=2
  wires:
  F I/P/1 -> Dot Product/1
  B I/P/1 -> Conjugate/1
  Conjugate/1 -> Dot Product/2
  Constant/1 -> Dot Product1/2
  Dot Product/1 -> Dot Product1/1
  Conjugate1/1 -> *K (K conjugate)/1
  Dot Product1/1 -> Subtract/2
  Subtract/1 -> K/1, Conjugate1/1
  K I/P/1 -> Subtract/1

== system FM_Bistatic_Radar_Full/Adaptive Filter/Gradiant Adaptive Lattice/50-Stage Lattice Predictor/Stage 34/K Update Equation ==
  F I/P : Inport
  B I/P : Inport  Port=2
  K I/P : Inport  Port=3
  Conjugate : Math  Operator=conj  SignedPower=on  RndMeth=Zero
  Conjugate1 : Math  Operator=conj  SignedPower=on  RndMeth=Zero
  Constant : Constant  Value=0.01
  Dot Product : DotProduct  OutDataTypeStr=Inherit: Inherit via internal rule
  Dot Product1 : DotProduct  OutDataTypeStr=Inherit: Inherit via internal rule
  Subtract : Sum  Inputs=+-
  *K (K conjugate) : Outport
  K : Outport  Port=2
  wires:
  F I/P/1 -> Dot Product/1
  B I/P/1 -> Conjugate/1
  Conjugate/1 -> Dot Product/2
  Constant/1 -> Dot Product1/2
  Dot Product/1 -> Dot Product1/1
  Conjugate1/1 -> *K (K conjugate)/1
  Dot Product1/1 -> Subtract/2
  Subtract/1 -> K/1, Conjugate1/1
  K I/P/1 -> Subtract/1

== system FM_Bistatic_Radar_Full/Adaptive Filter/Gradiant Adaptive Lattice/50-Stage Lattice Predictor/Stage 35/K Update Equation ==
  F I/P : Inport
  B I/P : Inport  Port=2
  K I/P : Inport  Port=3
  Conjugate : Math  Operator=conj  SignedPower=on  RndMeth=Zero
  Conjugate1 : Math  Operator=conj  SignedPower=on  RndMeth=Zero
  Constant : Constant  Value=0.01
  Dot Product : DotProduct  OutDataTypeStr=Inherit: Inherit via internal rule
  Dot Product1 : DotProduct  OutDataTypeStr=Inherit: Inherit via internal rule
  Subtract : Sum  Inputs=+-
  *K (K conjugate) : Outport
  K : Outport  Port=2
  wires:
  F I/P/1 -> Dot Product/1
  B I/P/1 -> Conjugate/1
  Conjugate/1 -> Dot Product/2
  Constant/1 -> Dot Product1/2
  Dot Product/1 -> Dot Product1/1
  Conjugate1/1 -> *K (K conjugate)/1
  Dot Product1/1 -> Subtract/2
  Subtract/1 -> K/1, Conjugate1/1
  K I/P/1 -> Subtract/1

== system FM_Bistatic_Radar_Full/Adaptive Filter/Gradiant Adaptive Lattice/50-Stage Lattice Predictor/Stage 36/K Update Equation ==
  F I/P : Inport
  B I/P : Inport  Port=2
  K I/P : Inport  Port=3
  Conjugate : Math  Operator=conj  SignedPower=on  RndMeth=Zero
  Conjugate1 : Math  Operator=conj  SignedPower=on  RndMeth=Zero
  Constant : Constant  Value=0.01
  Dot Product : DotProduct  OutDataTypeStr=Inherit: Inherit via internal rule
  Dot Product1 : DotProduct  OutDataTypeStr=Inherit: Inherit via internal rule
  Subtract : Sum  Inputs=+-
  *K (K conjugate) : Outport
  K : Outport  Port=2
  wires:
  F I/P/1 -> Dot Product/1
  B I/P/1 -> Conjugate/1
  Conjugate/1 -> Dot Product/2
  Constant/1 -> Dot Product1/2
  Dot Product/1 -> Dot Product1/1
  Conjugate1/1 -> *K (K conjugate)/1
  Dot Product1/1 -> Subtract/2
  Subtract/1 -> K/1, Conjugate1/1
  K I/P/1 -> Subtract/1

== system FM_Bistatic_Radar_Full/Adaptive Filter/Gradiant Adaptive Lattice/50-Stage Lattice Predictor/Stage 37/K Update Equation ==
  F I/P : Inport
  B I/P : Inport  Port=2
  K I/P : Inport  Port=3
  Conjugate : Math  Operator=conj  SignedPower=on  RndMeth=Zero
  Conjugate1 : Math  Operator=conj  SignedPower=on  RndMeth=Zero
  Constant : Constant  Value=0.01
  Dot Product : DotProduct  OutDataTypeStr=Inherit: Inherit via internal rule
  Dot Product1 : DotProduct  OutDataTypeStr=Inherit: Inherit via internal rule
  Subtract : Sum  Inputs=+-
  *K (K conjugate) : Outport
  K : Outport  Port=2
  wires:
  F I/P/1 -> Dot Product/1
  B I/P/1 -> Conjugate/1
  Conjugate/1 -> Dot Product/2
  Constant/1 -> Dot Product1/2
  Dot Product/1 -> Dot Product1/1
  Conjugate1/1 -> *K (K conjugate)/1
  Dot Product1/1 -> Subtract/2
  Subtract/1 -> K/1, Conjugate1/1
  K I/P/1 -> Subtract/1

== system FM_Bistatic_Radar_Full/Adaptive Filter/Gradiant Adaptive Lattice/50-Stage Lattice Predictor/Stage 38/K Update Equation ==
  F I/P : Inport
  B I/P : Inport  Port=2
  K I/P : Inport  Port=3
  Conjugate : Math  Operator=conj  SignedPower=on  RndMeth=Zero
  Conjugate1 : Math  Operator=conj  SignedPower=on  RndMeth=Zero
  Constant : Constant  Value=0.01
  Dot Product : DotProduct  OutDataTypeStr=Inherit: Inherit via internal rule
  Dot Product1 : DotProduct  OutDataTypeStr=Inherit: Inherit via internal rule
  Subtract : Sum  Inputs=+-
  *K (K conjugate) : Outport
  K : Outport  Port=2
  wires:
  F I/P/1 -> Dot Product/1
  B I/P/1 -> Conjugate/1
  Conjugate/1 -> Dot Product/2
  Constant/1 -> Dot Product1/2
  Dot Product/1 -> Dot Product1/1
  Conjugate1/1 -> *K (K conjugate)/1
  Dot Product1/1 -> Subtract/2
  Subtract/1 -> K/1, Conjugate1/1
  K I/P/1 -> Subtract/1

== system FM_Bistatic_Radar_Full/Adaptive Filter/Gradiant Adaptive Lattice/50-Stage Lattice Predictor/Stage 39/K Update Equation ==
  F I/P : Inport
  B I/P : Inport  Port=2
  K I/P : Inport  Port=3
  Conjugate : Math  Operator=conj  SignedPower=on  RndMeth=Zero
  Conjugate1 : Math  Operator=conj  SignedPower=on  RndMeth=Zero
  Constant : Constant  Value=0.01
  Dot Product : DotProduct  OutDataTypeStr=Inherit: Inherit via internal rule
  Dot Product1 : DotProduct  OutDataTypeStr=Inherit: Inherit via internal rule
  Subtract : Sum  Inputs=+-
  *K (K conjugate) : Outport
  K : Outport  Port=2
  wires:
  F I/P/1 -> Dot Product/1
  B I/P/1 -> Conjugate/1
  Conjugate/1 -> Dot Product/2
  Constant/1 -> Dot Product1/2
  Dot Product/1 -> Dot Product1/1
  Conjugate1/1 -> *K (K conjugate)/1
  Dot Product1/1 -> Subtract/2
  Subtract/1 -> K/1, Conjugate1/1
  K I/P/1 -> Subtract/1

== system FM_Bistatic_Radar_Full/Adaptive Filter/Gradiant Adaptive Lattice/50-Stage Lattice Predictor/Stage 4/K Update Equation ==
  F I/P : Inport
  B I/P : Inport  Port=2
  K I/P : Inport  Port=3
  Conjugate : Math  Operator=conj  SignedPower=on  RndMeth=Zero
  Conjugate1 : Math  Operator=conj  SignedPower=on  RndMeth=Zero
  Constant : Constant  Value=0.01
  Dot Product : DotProduct  OutDataTypeStr=Inherit: Inherit via internal rule
  Dot Product1 : DotProduct  OutDataTypeStr=Inherit: Inherit via internal rule
  Subtract : Sum  Inputs=+-
  *K (K conjugate) : Outport
  K : Outport  Port=2
  wires:
  F I/P/1 -> Dot Product/1
  B I/P/1 -> Conjugate/1
  Conjugate/1 -> Dot Product/2
  Constant/1 -> Dot Product1/2
  Dot Product/1 -> Dot Product1/1
  Conjugate1/1 -> *K (K conjugate)/1
  Dot Product1/1 -> Subtract/2
  Subtract/1 -> K/1, Conjugate1/1
  K I/P/1 -> Subtract/1

== system FM_Bistatic_Radar_Full/Adaptive Filter/Gradiant Adaptive Lattice/50-Stage Lattice Predictor/Stage 40/K Update Equation ==
  F I/P : Inport
  B I/P : Inport  Port=2
  K I/P : Inport  Port=3
  Conjugate : Math  Operator=conj  SignedPower=on  RndMeth=Zero
  Conjugate1 : Math  Operator=conj  SignedPower=on  RndMeth=Zero
  Constant : Constant  Value=0.01
  Dot Product : DotProduct  OutDataTypeStr=Inherit: Inherit via internal rule
  Dot Product1 : DotProduct  OutDataTypeStr=Inherit: Inherit via internal rule
  Subtract : Sum  Inputs=+-
  *K (K conjugate) : Outport
  K : Outport  Port=2
  wires:
  F I/P/1 -> Dot Product/1
  B I/P/1 -> Conjugate/1
  Conjugate/1 -> Dot Product/2
  Constant/1 -> Dot Product1/2
  Dot Product/1 -> Dot Product1/1
  Conjugate1/1 -> *K (K conjugate)/1
  Dot Product1/1 -> Subtract/2
  Subtract/1 -> K/1, Conjugate1/1
  K I/P/1 -> Subtract/1

== system FM_Bistatic_Radar_Full/Adaptive Filter/Gradiant Adaptive Lattice/50-Stage Lattice Predictor/Stage 41/K Update Equation ==
  F I/P : Inport
  B I/P : Inport  Port=2
  K I/P : Inport  Port=3
  Conjugate : Math  Operator=conj  SignedPower=on  RndMeth=Zero
  Conjugate1 : Math  Operator=conj  SignedPower=on  RndMeth=Zero
  Constant : Constant  Value=0.01
  Dot Product : DotProduct  OutDataTypeStr=Inherit: Inherit via internal rule
  Dot Product1 : DotProduct  OutDataTypeStr=Inherit: Inherit via internal rule
  Subtract : Sum  Inputs=+-
  *K (K conjugate) : Outport
  K : Outport  Port=2
  wires:
  F I/P/1 -> Dot Product/1
  B I/P/1 -> Conjugate/1
  Conjugate/1 -> Dot Product/2
  Constant/1 -> Dot Product1/2
  Dot Product/1 -> Dot Product1/1
  Conjugate1/1 -> *K (K conjugate)/1
  Dot Product1/1 -> Subtract/2
  Subtract/1 -> K/1, Conjugate1/1
  K I/P/1 -> Subtract/1

== system FM_Bistatic_Radar_Full/Adaptive Filter/Gradiant Adaptive Lattice/50-Stage Lattice Predictor/Stage 42/K Update Equation ==
  F I/P : Inport
  B I/P : Inport  Port=2
  K I/P : Inport  Port=3
  Conjugate : Math  Operator=conj  SignedPower=on  RndMeth=Zero
  Conjugate1 : Math  Operator=conj  SignedPower=on  RndMeth=Zero
  Constant : Constant  Value=0.01
  Dot Product : DotProduct  OutDataTypeStr=Inherit: Inherit via internal rule
  Dot Product1 : DotProduct  OutDataTypeStr=Inherit: Inherit via internal rule
  Subtract : Sum  Inputs=+-
  *K (K conjugate) : Outport
  K : Outport  Port=2
  wires:
  F I/P/1 -> Dot Product/1
  B I/P/1 -> Conjugate/1
  Conjugate/1 -> Dot Product/2
  Constant/1 -> Dot Product1/2
  Dot Product/1 -> Dot Product1/1
  Conjugate1/1 -> *K (K conjugate)/1
  Dot Product1/1 -> Subtract/2
  Subtract/1 -> K/1, Conjugate1/1
  K I/P/1 -> Subtract/1

== system FM_Bistatic_Radar_Full/Adaptive Filter/Gradiant Adaptive Lattice/50-Stage Lattice Predictor/Stage 43/K Update Equation ==
  F I/P : Inport
  B I/P : Inport  Port=2
  K I/P : Inport  Port=3
  Conjugate : Math  Operator=conj  SignedPower=on  RndMeth=Zero
  Conjugate1 : Math  Operator=conj  SignedPower=on  RndMeth=Zero
  Constant : Constant  Value=0.01
  Dot Product : DotProduct  OutDataTypeStr=Inherit: Inherit via internal rule
  Dot Product1 : DotProduct  OutDataTypeStr=Inherit: Inherit via internal rule
  Subtract : Sum  Inputs=+-
  *K (K conjugate) : Outport
  K : Outport  Port=2
  wires:
  F I/P/1 -> Dot Product/1
  B I/P/1 -> Conjugate/1
  Conjugate/1 -> Dot Product/2
  Constant/1 -> Dot Product1/2
  Dot Product/1 -> Dot Product1/1
  Conjugate1/1 -> *K (K conjugate)/1
  Dot Product1/1 -> Subtract/2
  Subtract/1 -> K/1, Conjugate1/1
  K I/P/1 -> Subtract/1

== system FM_Bistatic_Radar_Full/Adaptive Filter/Gradiant Adaptive Lattice/50-Stage Lattice Predictor/Stage 44/K Update Equation ==
  F I/P : Inport
  B I/P : Inport  Port=2
  K I/P : Inport  Port=3
  Conjugate : Math  Operator=conj  SignedPower=on  RndMeth=Zero
  Conjugate1 : Math  Operator=conj  SignedPower=on  RndMeth=Zero
  Constant : Constant  Value=0.01
  Dot Product : DotProduct  OutDataTypeStr=Inherit: Inherit via internal rule
  Dot Product1 : DotProduct  OutDataTypeStr=Inherit: Inherit via internal rule
  Subtract : Sum  Inputs=+-
  *K (K conjugate) : Outport
  K : Outport  Port=2
  wires:
  F I/P/1 -> Dot Product/1
  B I/P/1 -> Conjugate/1
  Conjugate/1 -> Dot Product/2
  Constant/1 -> Dot Product1/2
  Dot Product/1 -> Dot Product1/1
  Conjugate1/1 -> *K (K conjugate)/1
  Dot Product1/1 -> Subtract/2
  Subtract/1 -> K/1, Conjugate1/1
  K I/P/1 -> Subtract/1

== system FM_Bistatic_Radar_Full/Adaptive Filter/Gradiant Adaptive Lattice/50-Stage Lattice Predictor/Stage 45/K Update Equation ==
  F I/P : Inport
  B I/P : Inport  Port=2
  K I/P : Inport  Port=3
  Conjugate : Math  Operator=conj  SignedPower=on  RndMeth=Zero
  Conjugate1 : Math  Operator=conj  SignedPower=on  RndMeth=Zero
  Constant : Constant  Value=0.01
  Dot Product : DotProduct  OutDataTypeStr=Inherit: Inherit via internal rule
  Dot Product1 : DotProduct  OutDataTypeStr=Inherit: Inherit via internal rule
  Subtract : Sum  Inputs=+-
  *K (K conjugate) : Outport
  K : Outport  Port=2
  wires:
  F I/P/1 -> Dot Product/1
  B I/P/1 -> Conjugate/1
  Conjugate/1 -> Dot Product/2
  Constant/1 -> Dot Product1/2
  Dot Product/1 -> Dot Product1/1
  Conjugate1/1 -> *K (K conjugate)/1
  Dot Product1/1 -> Subtract/2
  Subtract/1 -> K/1, Conjugate1/1
  K I/P/1 -> Subtract/1

== system FM_Bistatic_Radar_Full/Adaptive Filter/Gradiant Adaptive Lattice/50-Stage Lattice Predictor/Stage 46/K Update Equation ==
  F I/P : Inport
  B I/P : Inport  Port=2
  K I/P : Inport  Port=3
  Conjugate : Math  Operator=conj  SignedPower=on  RndMeth=Zero
  Conjugate1 : Math  Operator=conj  SignedPower=on  RndMeth=Zero
  Constant : Constant  Value=0.01
  Dot Product : DotProduct  OutDataTypeStr=Inherit: Inherit via internal rule
  Dot Product1 : DotProduct  OutDataTypeStr=Inherit: Inherit via internal rule
  Subtract : Sum  Inputs=+-
  *K (K conjugate) : Outport
  K : Outport  Port=2
  wires:
  F I/P/1 -> Dot Product/1
  B I/P/1 -> Conjugate/1
  Conjugate/1 -> Dot Product/2
  Constant/1 -> Dot Product1/2
  Dot Product/1 -> Dot Product1/1
  Conjugate1/1 -> *K (K conjugate)/1
  Dot Product1/1 -> Subtract/2
  Subtract/1 -> K/1, Conjugate1/1
  K I/P/1 -> Subtract/1

== system FM_Bistatic_Radar_Full/Adaptive Filter/Gradiant Adaptive Lattice/50-Stage Lattice Predictor/Stage 47/K Update Equation ==
  F I/P : Inport
  B I/P : Inport  Port=2
  K I/P : Inport  Port=3
  Conjugate : Math  Operator=conj  SignedPower=on  RndMeth=Zero
  Conjugate1 : Math  Operator=conj  SignedPower=on  RndMeth=Zero
  Constant : Constant  Value=0.01
  Dot Product : DotProduct  OutDataTypeStr=Inherit: Inherit via internal rule
  Dot Product1 : DotProduct  OutDataTypeStr=Inherit: Inherit via internal rule
  Subtract : Sum  Inputs=+-
  *K (K conjugate) : Outport
  K : Outport  Port=2
  wires:
  F I/P/1 -> Dot Product/1
  B I/P/1 -> Conjugate/1
  Conjugate/1 -> Dot Product/2
  Constant/1 -> Dot Product1/2
  Dot Product/1 -> Dot Product1/1
  Conjugate1/1 -> *K (K conjugate)/1
  Dot Product1/1 -> Subtract/2
  Subtract/1 -> K/1, Conjugate1/1
  K I/P/1 -> Subtract/1

== system FM_Bistatic_Radar_Full/Adaptive Filter/Gradiant Adaptive Lattice/50-Stage Lattice Predictor/Stage 48/K Update Equation ==
  F I/P : Inport
  B I/P : Inport  Port=2
  K I/P : Inport  Port=3
  Conjugate : Math  Operator=conj  SignedPower=on  RndMeth=Zero
  Conjugate1 : Math  Operator=conj  SignedPower=on  RndMeth=Zero
  Constant : Constant  Value=0.01
  Dot Product : DotProduct  OutDataTypeStr=Inherit: Inherit via internal rule
  Dot Product1 : DotProduct  OutDataTypeStr=Inherit: Inherit via internal rule
  Subtract : Sum  Inputs=+-
  *K (K conjugate) : Outport
  K : Outport  Port=2
  wires:
  F I/P/1 -> Dot Product/1
  B I/P/1 -> Conjugate/1
  Conjugate/1 -> Dot Product/2
  Constant/1 -> Dot Product1/2
  Dot Product/1 -> Dot Product1/1
  Conjugate1/1 -> *K (K conjugate)/1
  Dot Product1/1 -> Subtract/2
  Subtract/1 -> K/1, Conjugate1/1
  K I/P/1 -> Subtract/1

== system FM_Bistatic_Radar_Full/Adaptive Filter/Gradiant Adaptive Lattice/50-Stage Lattice Predictor/Stage 49/K Update Equation ==
  F I/P : Inport
  B I/P : Inport  Port=2
  K I/P : Inport  Port=3
  Conjugate : Math  Operator=conj  SignedPower=on  RndMeth=Zero
  Conjugate1 : Math  Operator=conj  SignedPower=on  RndMeth=Zero
  Constant : Constant  Value=0.01
  Dot Product : DotProduct  OutDataTypeStr=Inherit: Inherit via internal rule
  Dot Product1 : DotProduct  OutDataTypeStr=Inherit: Inherit via internal rule
  Subtract : Sum  Inputs=+-
  *K (K conjugate) : Outport
  K : Outport  Port=2
  wires:
  F I/P/1 -> Dot Product/1
  B I/P/1 -> Conjugate/1
  Conjugate/1 -> Dot Product/2
  Constant/1 -> Dot Product1/2
  Dot Product/1 -> Dot Product1/1
  Conjugate1/1 -> *K (K conjugate)/1
  Dot Product1/1 -> Subtract/2
  Subtract/1 -> K/1, Conjugate1/1
  K I/P/1 -> Subtract/1
